simulink model "snimanjeodziva"  (R2013a)
settings: Solver=ode3  StartTime=0.0  StopTime=inf  FixedStep=0.001  RelTol=1e-3
undefined symbols (not defined in the file): analoginput
libraries: daqlib x2
settings Model: Creator=student  LastModifiedBy=student

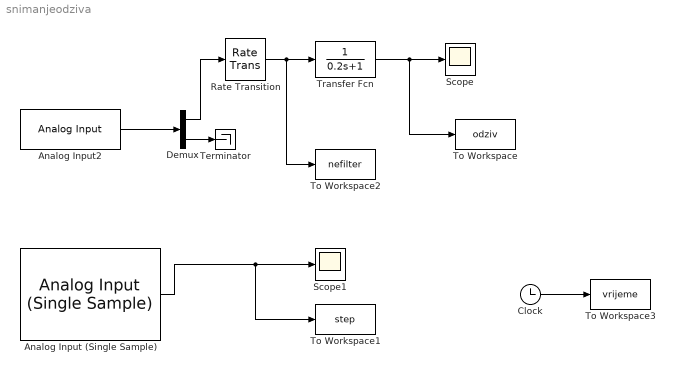
== system snimanjeodziva ==
  Analog Input (Single Sample) : daqlib/Analog Input (Single Sample)  DeviceMenu=nidaq Dev1 (PCI-6024E)  Device=nidaq Dev1 (PCI-6024E)  ObjConstructor=analoginput('nidaq','Dev1')  InputType=SingleEnded  NChannelsSelected=1  Channels=0$0$$1$#0$1$$1$#0$2$$1$#0$3$$1$#1$4$$1$#0$5$$1$#0$6$$1$#0$7$$1$#0$8$$1$#0$9$$1$#0$10$$1$#0$11$$1$#0$12$$1$#0$13$$1$#0$14$$1$#0$15$$1$#  NPorts=1 per hardware channel  BlockSampleTime=1
  Analog Input2 : daqlib/Analog Input  AcqMode=0  DeviceMenu=nidaq Dev1 (PCI-6024E)  Device=nidaq Dev1 (PCI-6024E)  ObjConstructor=analoginput('nidaq','Dev1')  SampleRate=1000  ActualRate=1000  SamplesPerFrame=2  InputType=SingleEnded  NChannelsSelected=1  Channels=0$0$$1$#0$1$$1$#0$2$$1$#0$3$$1$#0$4$$1$#0$5$$1$#1$6$$1$#0$7$$1$#0$8$$1$#0$9$$1$#0$10$$1$#0$11$$1$#0$12$$1$#0$13$$1$#0$14$$1$#0$15$$1$#  NPorts=1 per hardware channel  DataType=double
      settings: SignalType=Sample-based
  Clock : Clock
  Demux : Demux  Outputs=2
  Rate Transition : RateTransition
  Scope : Scope
  Scope1 : Scope
  Terminator : Terminator
  To Workspace : ToWorkspace  VariableName=odziv  SampleTime=-1
  To Workspace1 : ToWorkspace  VariableName=step  SampleTime=-1
  To Workspace2 : ToWorkspace  VariableName=nefilter  SampleTime=-1
  To Workspace3 : ToWorkspace  VariableName=vrijeme  SampleTime=-1
  Transfer Fcn : TransferFcn  Denominator=[0.2 1]
  wires:
  Analog Input (Single Sample)/1 -> To Workspace1/1, Scope1/1
  Analog Input2/1 -> Demux/1
  Demux/2 -> Terminator/1
  Transfer Fcn/1 -> To Workspace/1, Scope/1
  Rate Transition/1 -> To Workspace2/1, Transfer Fcn/1
  Demux/1 -> Rate Transition/1
  Clock/1 -> To Workspace3/1
